simulink model "cantp"  (R2020a)
settings: Solver=VariableStepAuto  StartTime=0.0  StopTime=inf  RelTol=1e-3
InitFcn:
  | messagePeriod=1.0;%must be greater than 5ms.
  | 
  | Fsquare=1;
  | squareTs=0.01/Fsquare;
  | squareSamplesPerPeriod=fix(1/Fsquare/squareTs);
  | squareSamplesPerPulseWidth=fix(squareSamplesPerPeriod/2);
  | squareAmplitude=1;
  | 
  | Fsinus=0.05;
  | sinusTs=0.01/Fsinus;
  | sinusSamplesPerPeriod=fix(1/Fsinus/sinusTs);
  | sinusAmplitude=100;
  | rxCANSampleTime=0.01;
undefined symbols (not defined in the file): canChannel
libraries: canlib x14, canmsglib x14, simulink x6
(part 2 of 2)

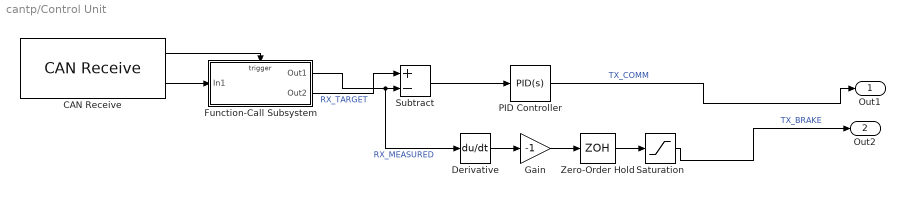
== system cantp/Control Unit ==
  CAN Receive : canlib/CAN Receive  BlockHandle=548.0002  Device=MathWorks Virtual 1 (Channel 1)  DeviceMenu=MathWorks Virtual 1 (Channel 1)  ObjConstructor=canChannel('MathWorks', 'Virtual 1', 1)  EnableStandardIDsFilter=off  StdIDsCombo=Allow only  StandardIDs=[1 3]  EnableExtendedIDsFilter=off  ExtIDsCombo=Allow all  ExtendedIDs=0  SampleTime=0.001  MsgsPerTimestep=all  InternalFilterUpdateStatus=on  BusOutput=off
      settings: SourceProductBaseCode=VN
  Derivative : Derivative
  Function-Call Subsystem : Subsystem  TreatAsAtomicUnit=on
  Gain : Gain  Gain=-1
  PID Controller : simulink/Continuous/PID Controller  Controller=PID  Form=Parallel  TimeDomain=Continuous-time  UseExternalTs=off  SampleTime=-1  IntegratorMethod=Forward Euler  ControllerParametersSource=internal  P=1  I=0.5  D=0  UseFilter=on  N=0.2  TunerSelectOption=Transfer Function Based (PID Tuner App)  InitialConditionSource=internal  InitialConditionForIntegrator=0  InitialConditionForFilter=0  DifferentiatorICPrevScaledInput=0  ExternalReset=none  TrackingMode=off  Kt=1  LimitOutput=off  UpperSaturationLimit=inf  LowerSaturationLimit=-inf  LinearizeAsGain=on  AntiWindupMode=none  Kb=1  POutMin=[]  POutMax=[]  IOutMin=[]  IOutMax=[]  DOutMin=[]  DOutMax=[]  NOutMin=[]  NOutMax=[]  SumOutMin=[]  SumOutMax=[]  SaturationOutMin=[]  SaturationOutMax=[]  PParamMin=[]  PParamMax=[]  IParamMin=[]  IParamMax=[]  DParamMin=[]  DParamMax=[]  NParamMin=[]  NParamMax=[]  KbParamMin=[]  KbParamMax=[]  KtParamMin=[]  KtParamMax=[]  KbOutMin=[]  KbOutMax=[]  KtOutMin=[]  KtOutMax=[]  IntegratorOutMin=[]  IntegratorOutMax=[]  FilterOutMin=[]  FilterOutMax=[]  SumI1OutMin=[]  SumI1OutMax=[]  SumI2OutMin=[]  SumI2OutMax=[]  SumI3OutMin=[]  SumI3OutMax=[]  SumI4OutMin=[]  SumI4OutMax=[]  SumDOutMin=[]  SumDOutMax=[]  DifferentiatorOutMin=[]  DifferentiatorOutMax=[]  FilterDiffOutCoefMin=[]  FilterDiffOutCoefMax=[]  ReciprocalOutMin=[]  ReciprocalOutMax=[]  SumDenOutMin=[]  SumDenOutMax=[]  SumNumOutMin=[]  SumNumOutMax=[]  DivideOutMin=[]  DivideOutMax=[]  UdiffTsProdOutMin=[]  UdiffTsProdOutMax=[]  NTsProdOutMin=[]  NTsProdOutMax=[]  UintegralTsProdOutMin=[]  UintegralTsProdOutMax=[]  UngainTsProdOutMin=[]  UngainTsProdOutMax=[]  IntegratorContinuousStateAttributes=''  IntegratorStateMustResolveToSignalObject=off  IntegratorRTWStateStorageClass=Auto  FilterContinuousStateAttributes=''  FilterStateMustResolveToSignalObject=off  FilterRTWStateStorageClass=Auto  ParallelPVariant=InternalParameters  IdealPVariant=Disabled  IVariant=InternalParameters  DVariant=InternalParameters  IntegratorVariant=Continuous  SatVariant=Disabled  AWVariant=Passthrough  PCopyVariant=Disabled  TRVariant=Disabled  FdbkBlocksVariant=Forward  IdealPFdbkVariant=Disabled  SatFdbkVariant=Disabled  DerivativeFilterVariant=ContFilter  NVariant=InternalParameters  NCopyVariant=Disabled  FilterICVariant=InternalICsFilter  IntegratorICVariant=InternalICs  ExternalResetVariant=Disabled  TRSumVariant=Passthrough  SumFdbkVariant=Disabled  SumVariant=Sum_PID  TsampFilterVariant=InternalTs  TsampNgainVariant=Passthrough  TsampIntegralVariant=Passthrough
  Saturation : Saturate  UpperLimit=1  LowerLimit=-1
  Subtract : Sum  Inputs=+-
  Zero-Order Hold : ZeroOrderHold
  Out1 : Outport
  Out2 : Outport  Port=2
  wires:
  Subtract/1 -> PID Controller/1
  Gain/1 -> Zero-Order Hold/1
  Derivative/1 -> Gain/1
  Saturation/1 -> Out2/1  "TX_BRAKE"
  Zero-Order Hold/1 -> Saturation/1
  Function-Call Subsystem/1(Out1) -> Derivative/1, Subtract/2  "RX_MEASURED"
  CAN Receive/2 -> Function-Call Subsystem/1(In1)
  CAN Receive/1 -> Function-Call Subsystem/Trigger
  PID Controller/1 -> Out1/1  "TX_COMM"
  Function-Call Subsystem/2(Out2) -> Subtract/1  "RX_TARGET"

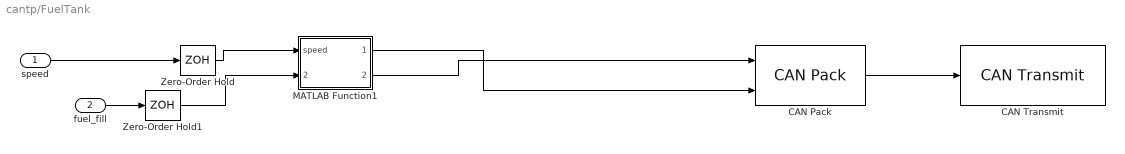
== system cantp/FuelTank ==
  speed : Inport
  fuel_fill : Inport  Port=2
  CAN Pack : canmsglib/CAN Pack  MsgList=(none)  MsgName=Fuel Msg  MsgIDType=Standard (11-bit identifier)  MsgIdentifier=5  MsgLength=2  Remote=off  ApplyMinMax=off  BusOutput=off  SignalInfo={ 'ETAT', '0', '1', 'LE', 'unsigned', 'Standard', '0', '1', '0', '0', '1'; 'LEVEL', '1', '8', 'LE', 'unsigned', 'Standard', '0', '1', '0', '-Inf', 'Inf' }
      settings: SourceProductBaseCode=ME,XP,VN  DataFormat=manually specified signals
  CAN Transmit : canlib/CAN Transmit  BlockHandle=593.0002  Device=MathWorks Virtual 1 (Channel 1)  DeviceMenu=MathWorks Virtual 1 (Channel 1)  ObjConstructor=canChannel('MathWorks', 'Virtual 1', 1)  EnableEventTransmit=off  EnablePeriodicTransmit=on  MessagePeriod=0.025
      settings: SourceProductBaseCode=VN
  MATLAB Function1 : MATLAB Function  TreatAsAtomicUnit=on
  Zero-Order Hold : ZeroOrderHold  SampleTime=0.01
  Zero-Order Hold1 : ZeroOrderHold  SampleTime=0.01
  wires:
  speed/1 -> Zero-Order Hold/1
  fuel_fill/1 -> Zero-Order Hold1/1
  Zero-Order Hold/1 -> MATLAB Function1/1(speed)
  CAN Pack/1 -> CAN Transmit/1
  MATLAB Function1/1(fuel_level) -> CAN Pack/2
  Zero-Order Hold1/1 -> MATLAB Function1/2(fuel_fill)
  MATLAB Function1/2(led_status) -> CAN Pack/1

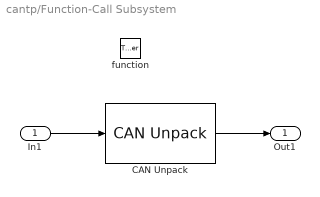
== system cantp/Function-Call Subsystem ==
  In1 : Inport
  function : TriggerPort  TriggerType=function-call  VariantControl=(inherit)
  CAN Unpack : canmsglib/CAN Unpack  MsgList=(none)  MsgName=VM message  MsgIDType=Standard (11-bit identifier)  MsgIdentifier=1  MsgLength=4  SignalInfo={ 'VM', '0', '8', 'LE', 'unsigned', 'Standard', '0', '1', '0', '-Inf', 'Inf' }  IDPort=off  TimestampPort=off  ErrorPort=off  RemotePort=off  LengthPort=off  StatusPort=off  ApplyMinMax=off
      settings: SourceProductBaseCode=ME,XP,VN
  Out1 : Outport
  wires:
  In1/1 -> CAN Unpack/1
  CAN Unpack/1 -> Out1/1

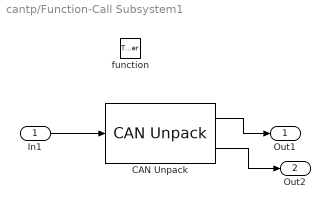
== system cantp/Function-Call Subsystem1 ==
  In1 : Inport
  function : TriggerPort  TriggerType=function-call  VariantControl=(inherit)
  CAN Unpack : canmsglib/CAN Unpack  MsgList=(none)  MsgName=DASHBOARD msg  MsgIDType=Standard (11-bit identifier)  MsgIdentifier=2  MsgLength=1  SignalInfo={ 'LEDRIGHT', '0', '1', 'LE', 'unsigned', 'Standard', '0', '1', '0', '0', '1'; 'LEDLEFT', '1', '1', 'LE', 'unsigned', 'Standard', '0', '1', '0', '0', '1' }  IDPort=off  TimestampPort=off  ErrorPort=off  RemotePort=off  LengthPort=off  StatusPort=off  ApplyMinMax=off
      settings: SourceProductBaseCode=ME,XP,VN
  Out1 : Outport
  Out2 : Outport  Port=2
  wires:
  In1/1 -> CAN Unpack/1
  CAN Unpack/1 -> Out1/1
  CAN Unpack/2 -> Out2/1

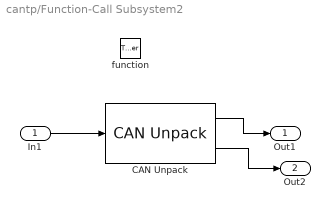
== system cantp/Function-Call Subsystem2 ==
  In1 : Inport
  function : TriggerPort  TriggerType=function-call  VariantControl=(inherit)
  CAN Unpack : canmsglib/CAN Unpack  MsgList=(none)  MsgName=DASHBOARD msg  MsgIDType=Standard (11-bit identifier)  MsgIdentifier=2  MsgLength=1  SignalInfo={ 'LEDRIGHT', '0', '1', 'LE', 'unsigned', 'Standard', '0', '1', '0', '0', '1'; 'LEDLEFT', '1', '1', 'LE', 'unsigned', 'Standard', '0', '1', '0', '0', '1' }  IDPort=off  TimestampPort=off  ErrorPort=off  RemotePort=off  LengthPort=off  StatusPort=off  ApplyMinMax=off
      settings: SourceProductBaseCode=ME,XP,VN
  Out1 : Outport
  Out2 : Outport  Port=2
  wires:
  In1/1 -> CAN Unpack/1
  CAN Unpack/1 -> Out1/1
  CAN Unpack/2 -> Out2/1

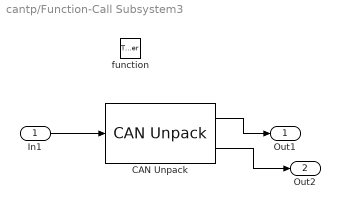
== system cantp/Function-Call Subsystem3 ==
  In1 : Inport
  function : TriggerPort  TriggerType=function-call  VariantControl=(inherit)
  CAN Unpack : canmsglib/CAN Unpack  MsgList=(none)  MsgName=VM message  MsgIDType=Standard (11-bit identifier)  MsgIdentifier=5  MsgLength=2  SignalInfo={ 'ETAT', '0', '1', 'LE', 'unsigned', 'Standard', '0', '1', '0', '0', '1'; 'LEVEL', '1', '8', 'LE', 'unsigned', 'Standard', '0', '1', '0', '-Inf', 'Inf' }  IDPort=off  TimestampPort=off  ErrorPort=off  RemotePort=off  LengthPort=off  StatusPort=off  ApplyMinMax=off
      settings: SourceProductBaseCode=ME,XP,VN
  Out1 : Outport
  Out2 : Outport  Port=2
  wires:
  In1/1 -> CAN Unpack/1
  CAN Unpack/1 -> Out1/1
  CAN Unpack/2 -> Out2/1

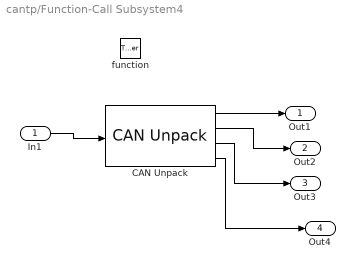
== system cantp/Function-Call Subsystem4 ==
  In1 : Inport
  function : TriggerPort  TriggerType=function-call  VariantControl=(inherit)
  CAN Unpack : canmsglib/CAN Unpack  MsgList=(none)  MsgName=SETTING message  MsgIDType=Standard (11-bit identifier)  MsgIdentifier=6  MsgLength=1  SignalInfo={ 'ABS', '0', '1', 'LE', 'unsigned', 'Standard', '0', '1', '0', '0', '1'; 'ESP', '1', '1', 'LE', 'unsigned', 'Standard', '0', '1', '0', '0', '1'; 'ECONOMIE', '2', '1', 'LE', 'unsigned', 'Standard', '0', '1', '0', '0', '1'; 'STABILIT', '3', '1', 'LE', 'unsigned', 'Standard', '0', '1', '0', '0', '1' }  IDPort=off  TimestampPort=off  ErrorPort=off  RemotePort=off  LengthPort=off  StatusPort=off  ApplyMinMax=off
      settings: SourceProductBaseCode=ME,XP,VN
  Out1 : Outport
  Out2 : Outport  Port=2
  Out3 : Outport  Port=3
  Out4 : Outport  Port=4
  wires:
  In1/1 -> CAN Unpack/1
  CAN Unpack/1 -> Out1/1
  CAN Unpack/2 -> Out2/1
  CAN Unpack/3 -> Out3/1
  CAN Unpack/4 -> Out4/1

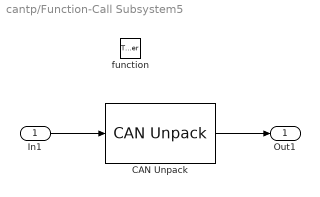
== system cantp/Function-Call Subsystem5 ==
  In1 : Inport
  function : TriggerPort  TriggerType=function-call  VariantControl=(inherit)
  CAN Unpack : canmsglib/CAN Unpack  MsgList=(none)  MsgName=VM message  MsgIDType=Standard (11-bit identifier)  MsgIdentifier=7  MsgLength=1  SignalInfo={ 'ETAT', '0', '1', 'LE', 'unsigned', 'Standard', '0', '1', '0', '0', '1' }  IDPort=off  TimestampPort=off  ErrorPort=off  RemotePort=off  LengthPort=off  StatusPort=off  ApplyMinMax=off
      settings: SourceProductBaseCode=ME,XP,VN
  Out1 : Outport
  wires:
  In1/1 -> CAN Unpack/1
  CAN Unpack/1 -> Out1/1

== system cantp/Push Button ==

== system cantp/Push Button1 ==

== system cantp/Push Button2 ==

== system cantp/Push Button3 ==

== system cantp/Rotary Switch1 ==

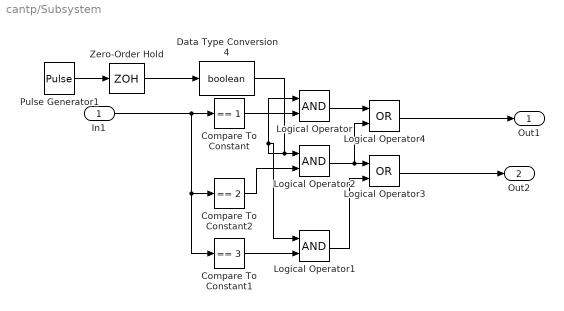
== system cantp/Subsystem ==
  In1 : Inport
  Compare To Constant : simulink/Logic and Bit Operations/Compare To Constant  relop===  const=1  OutDataTypeStr=boolean
  Compare To Constant1 : simulink/Logic and Bit Operations/Compare To Constant  relop===  const=3  OutDataTypeStr=boolean
  Compare To Constant2 : simulink/Logic and Bit Operations/Compare To Constant  relop===  const=2  OutDataTypeStr=boolean
  Data Type Conversion4 : DataTypeConversion  OutDataTypeStr=boolean
  Logical Operator : Logic  OutDataTypeStr=boolean
  Logical Operator1 : Logic  OutDataTypeStr=boolean
  Logical Operator2 : Logic  OutDataTypeStr=boolean
  Logical Operator3 : Logic  Operator=OR  OutDataTypeStr=boolean
  Logical Operator4 : Logic  Operator=OR  OutDataTypeStr=boolean
  Pulse Generator1 : DiscretePulseGenerator  PulseType=Time based  PulseWidth=50  SampleTime=0.1  VectorParams1D=off
  Zero-Order Hold : ZeroOrderHold  SampleTime=0.01
  Out1 : Outport  VectorParamsAs1DForOutWhenUnconnected=off
  Out2 : Outport  Port=2  VectorParamsAs1DForOutWhenUnconnected=off
  wires:
  Compare To Constant2/1 -> Logical Operator2/2
  Data Type Conversion4/1 -> Logical Operator/1, Logical Operator1/1, Logical Operator2/1
  Compare To Constant1/1 -> Logical Operator1/2
  Compare To Constant/1 -> Logical Operator/2
  Logical Operator1/1 -> Logical Operator3/2
  Logical Operator/1 -> Logical Operator4/1
  Logical Operator2/1 -> Logical Operator3/1, Logical Operator4/2
  In1/1 -> Compare To Constant1/1, Compare To Constant2/1, Compare To Constant/1
  Pulse Generator1/1 -> Zero-Order Hold/1
  Logical Operator4/1 -> Out1/1
  Logical Operator3/1 -> Out2/1
  Zero-Order Hold/1 -> Data Type Conversion4/1

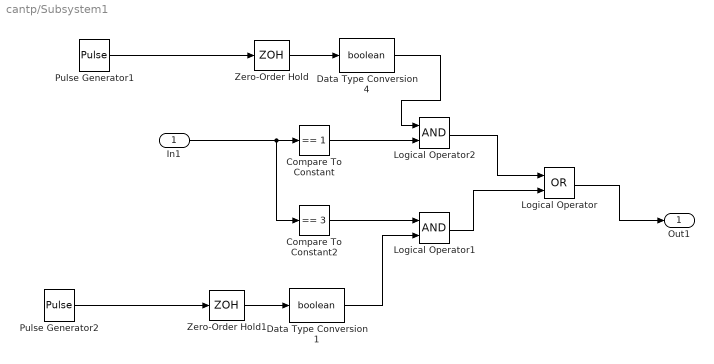
== system cantp/Subsystem1 ==
  In1 : Inport
  Compare To Constant : simulink/Logic and Bit Operations/Compare To Constant  relop===  const=1  OutDataTypeStr=boolean
  Compare To Constant2 : simulink/Logic and Bit Operations/Compare To Constant  relop===  const=3  OutDataTypeStr=boolean
  Data Type Conversion1 : DataTypeConversion  OutDataTypeStr=boolean
  Data Type Conversion4 : DataTypeConversion  OutDataTypeStr=boolean
  Logical Operator : Logic  Operator=OR  AllPortsSameDT=off  OutDataTypeStr=boolean
  Logical Operator1 : Logic  OutDataTypeStr=boolean
  Logical Operator2 : Logic  OutDataTypeStr=boolean
  Pulse Generator1 : DiscretePulseGenerator  PulseType=Time based  Period=10  PulseWidth=50  SampleTime=0.1  VectorParams1D=off
  Pulse Generator2 : DiscretePulseGenerator  PulseType=Time based  Period=5  PulseWidth=40  SampleTime=0.1  VectorParams1D=off
  Zero-Order Hold : ZeroOrderHold  SampleTime=0.01
  Zero-Order Hold1 : ZeroOrderHold  SampleTime=-1
  Out1 : Outport
  wires:
  In1/1 -> Compare To Constant2/1, Compare To Constant/1
  Compare To Constant2/1 -> Logical Operator1/1
  Compare To Constant/1 -> Logical Operator2/2
  Data Type Conversion4/1 -> Logical Operator2/1
  Data Type Conversion1/1 -> Logical Operator1/2
  Pulse Generator2/1 -> Zero-Order Hold1/1
  Logical Operator2/1 -> Logical Operator/1
  Logical Operator1/1 -> Logical Operator/2
  Logical Operator/1 -> Out1/1
  Zero-Order Hold1/1 -> Data Type Conversion1/1
  Zero-Order Hold/1 -> Data Type Conversion4/1
  Pulse Generator1/1 -> Zero-Order Hold/1

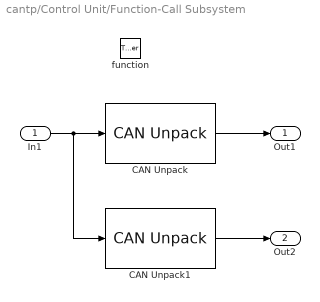
== system cantp/Control Unit/Function-Call Subsystem ==
  In1 : Inport
  function : TriggerPort  TriggerType=function-call  VariantControl=(inherit)
  CAN Unpack : canmsglib/CAN Unpack  MsgList=(none)  MsgName=VM message  MsgIDType=Standard (11-bit identifier)  MsgIdentifier=1  MsgLength=4  SignalInfo={ 'VM', '0', '8', 'LE', 'unsigned', 'Standard', '0', '1', '0', '-Inf', 'Inf' }  IDPort=off  TimestampPort=off  ErrorPort=off  RemotePort=off  LengthPort=off  StatusPort=off  ApplyMinMax=off
      settings: SourceProductBaseCode=ME,XP,VN
  CAN Unpack1 : canmsglib/CAN Unpack  MsgList=(none)  MsgName=VM message  MsgIDType=Standard (11-bit identifier)  MsgIdentifier=3  MsgLength=2  SignalInfo={ 'VM', '0', '8', 'LE', 'unsigned', 'Standard', '0', '1', '0', '0', '255' }  IDPort=off  TimestampPort=off  ErrorPort=off  RemotePort=off  LengthPort=off  StatusPort=off  ApplyMinMax=off
      settings: SourceProductBaseCode=ME,XP,VN
  Out1 : Outport
  Out2 : Outport  Port=2
  wires:
  CAN Unpack/1 -> Out1/1
  In1/1 -> CAN Unpack1/1, CAN Unpack/1
  CAN Unpack1/1 -> Out2/1

== matlab function cantp/FuelTank/MATLAB Function1 ==
  data: speed input; fuel_fill input; fuel_level output; led_status output
function [fuel_level, led_status] = car_fuel_model(speed, fuel_fill)
    persistent initial_fuel last_speed last_time max_fuel;
    max_speed = 240; % Maximum speed
    
    % Initialize max_fuel if not defined
    if isempty(max_fuel)
        max_fuel = 1; % Set initial maximum fuel capacity
    end
    
    % Define initial fuel if not defined
    if isempty(initial_fuel)
        initial_fuel = 0; % Set initial fuel to 0
        last_speed = speed; % Initialize last_speed
        last_time = tic; % Initialize last_time using tic
    end
    
    % Calculate time elapsed since last call
    current_time = toc(last_time);
    elapsed_time = current_time; % Use current_time directly
    
    % If fuel fill exceeds current max fuel, update max fuel
    if fuel_fill > max_fuel
        max_fuel = fuel_fill;
    end
    
    % If speed is 0, gradually add fuel fill to initial fuel
    if speed == 0
        % Calculate the fuel to add based on the time elapsed
        fuel_to_add = fuel_fill * 0.1 * elapsed_time; % Using a fixed rate
        
        % Increment the initial fuel
        initial_fuel = initial_fuel + fuel_to_add;
    else
        % Calculate the fuel consumption based on speed and time elapsed
        fuel_consumption = speed * 0.01 * elapsed_time;
        
        % Reduce the fuel level by the calculated fuel consumption rate
        initial_fuel = initial_fuel - fuel_consumption;
        
        % Ensure fuel level doesn't go below 0
        initial_fuel = max(initial_fuel, 0); % Use max function
    end
    
    % Ensure fuel level doesn't exceed the maximum capacity chosen by the slider
    initial_fuel = min(initial_fuel, max_fuel); % Use min function
    
    % Update last_speed and last_time for the next iteration
    last_speed = speed;
    last_time = tic; % Update last_time using tic
    
    % Output fuel level
    fuel_level = initial_fuel; 
    
    % Determine LED status
    if initial_fuel < 20
        led_status = 1; % LED is on
    else
        led_status = 0; % LED is off
    end
end
